simulink model "rfpsc_single"  (R2023b)
settings: Solver=VariableStepAuto  StartTime=0.0  StopTime=.5  RelTol=1e-3
undefined symbols (not defined in the file): f_sw, kpp, L_f, L_g, R_a, R_L, T_s, U_dc, u_gN, w_b, w_g
libraries: simulink x1
settings Model: Creator=maatt  LastModifiedBy=chowd
settings DataIOCC: ReturnWorkspaceOutputs=off

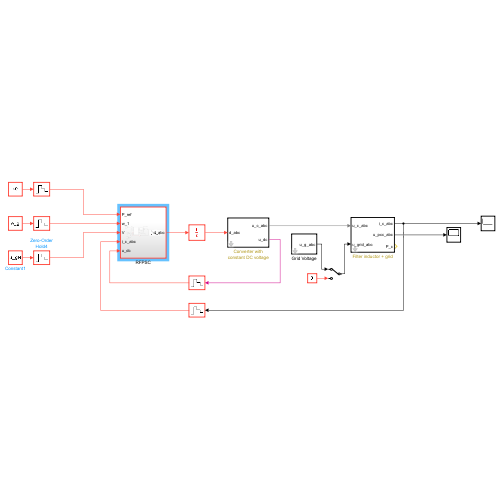
[thumbnail: Simulink's stored preview of the top-level diagram]
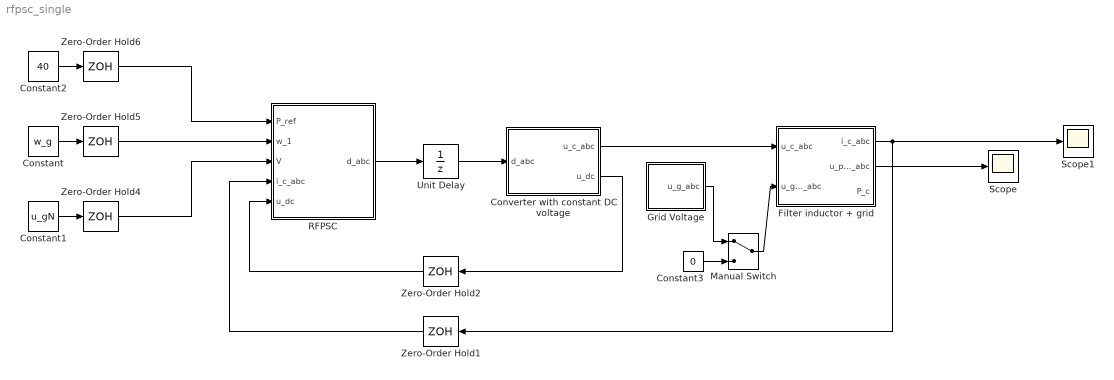
== system rfpsc_single ==
  Constant : Constant  Value=w_g  SampleTime=T_s
  Constant1 : Constant  Value=u_gN  SampleTime=T_s
  Constant2 : Constant  Value=40  SampleTime=T_s
  Constant3 : Constant  Value=0  SampleTime=T_s
  "Converter with constant DC voltage " : Subsystem  mask{f_sw=f_sw, u_dc=U_dc}
      mask prompts: f_sw "Switching frequency (Hz)"; u_dc "DC-bus voltage (V)"
      mask init:
      | T_s = 1/(2*f_sw);
  Filter inductor + grid : Subsystem  mask{L_f=L_f, L_g=L_g, R_L=R_L}
      mask prompts: L_f "Filter inductance (H)"; L_g "Grid inductance (H)"; R_L "Series resistance (ohm)"
  Grid Voltage : Subsystem  mask{U_g=u_gN, angle=0}
      mask prompts: U_g "Phase-voltage"; angle "Shift the phases of voltages"
  Manual Switch : ManualSwitch
  RFPSC : Subsystem
  Scope : Scope
  Scope1 : Scope
  Unit Delay : UnitDelay  SampleTime=T_s  HasFrameUpgradeWarning=on
  Zero-Order Hold{1..2,4..6} (5 alike) : ZeroOrderHold  SampleTime=T_s
  wires:
  "Converter with constant DC voltage "/2(u_dc) -> Zero-Order Hold2/1
  Constant/1 -> Zero-Order Hold5/1
  Constant1/1 -> Zero-Order Hold4/1
  Unit Delay/1 -> "Converter with constant DC voltage "/1(d_abc)
  Zero-Order Hold1/1 -> RFPSC/4(i_c_abc)
  Zero-Order Hold4/1 -> RFPSC/3(V)
  Zero-Order Hold2/1 -> RFPSC/5(u_dc)
  Constant2/1 -> Zero-Order Hold6/1
  Filter inductor + grid/1(i_c_abc) -> Scope1/1, Zero-Order Hold1/1
  Filter inductor + grid/2(u_pcc_abc) -> Scope/1
  Zero-Order Hold6/1 -> RFPSC/1(P_ref)
  Zero-Order Hold5/1 -> RFPSC/2(w_1)
  RFPSC/1(d_abc) -> Unit Delay/1
  Constant3/1 -> Manual Switch/2
  Manual Switch/1 -> Filter inductor + grid/2(u_grid_abc)
  "Converter with constant DC voltage "/1(u_c_abc) -> Filter inductor + grid/1(u_c_abc)
  Grid Voltage/1(u_g_abc) -> Manual Switch/1

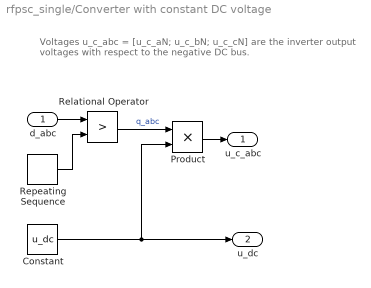
== system rfpsc_single/Converter with constant DC voltage  ==
  note: Voltages u_c_abc = [u_c_aN; u_c_bN; u_c_cN] are the inverter
      | output voltages with respect to the negative DC bus.
  d_abc : Inport
  Constant : Constant  Value=u_dc
  Product : Product
  Relational Operator : RelationalOperator  Operator=>  OutDataTypeStr='double'  InputSameDT=off
  Repeating Sequence : simulink/Sources/Repeating Sequence  rep_seq_t=[0 1 2]*T_s  rep_seq_y=[1 0 1]
  u_c_abc : Outport
  u_dc : Outport  Port=2
  wires:
  Repeating Sequence/1 -> Relational Operator/2
  d_abc/1 -> Relational Operator/1
  Product/1 -> u_c_abc/1
  Relational Operator/1 -> Product/1  "q_abc"
  Constant/1 -> Product/2, u_dc/1

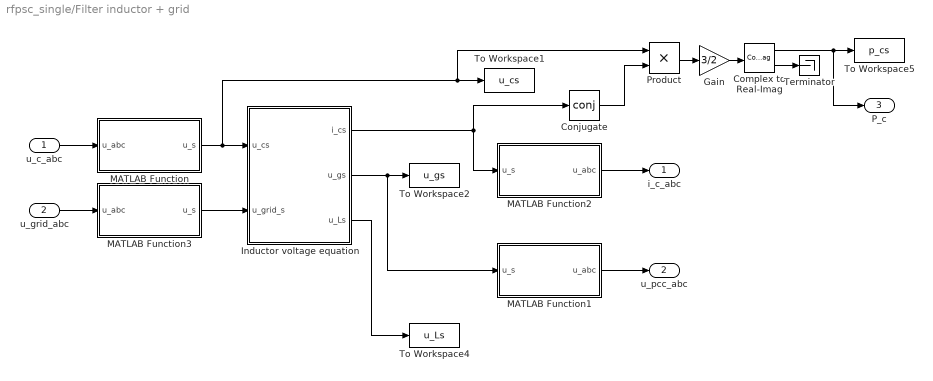
== system rfpsc_single/Filter inductor + grid ==
  u_c_abc : Inport
  u_grid_abc : Inport  Port=2
  Complex to Real-Imag : ComplexToRealImag
  Conjugate : Math  Operator=conj  SignedPower=on  RndMeth=Zero
  Gain : Gain  Gain=3/2
  Inductor voltage equation : Subsystem
  MATLAB Function : MATLAB Function  TreatAsAtomicUnit=on
  MATLAB Function1 : MATLAB Function  TreatAsAtomicUnit=on
  MATLAB Function2 : MATLAB Function  TreatAsAtomicUnit=on
  MATLAB Function3 : MATLAB Function  TreatAsAtomicUnit=on
  Product : Product
  Terminator : Terminator
  To Workspace1 : ToWorkspace  VariableName=u_cs  SaveFormat=Timeseries
  To Workspace2 : ToWorkspace  VariableName=u_gs  SaveFormat=Timeseries
  To Workspace4 : ToWorkspace  VariableName=u_Ls  SaveFormat=Timeseries
  To Workspace5 : ToWorkspace  VariableName=p_cs  SaveFormat=Timeseries
  i_c_abc : Outport
  u_pcc_abc : Outport  Port=2
  P_c : Outport  Port=3
  wires:
  u_c_abc/1 -> MATLAB Function/1(u_abc)
  Inductor voltage equation/1(i_cs) -> MATLAB Function2/1(u_s), Conjugate/1
  MATLAB Function2/1(u_abc) -> i_c_abc/1
  MATLAB Function/1(u_s) -> Inductor voltage equation/1(u_cs), Product/1, To Workspace1/1
  Inductor voltage equation/2(u_gs) -> MATLAB Function1/1(u_s), To Workspace2/1
  Inductor voltage equation/3(u_Ls) -> To Workspace4/1
  MATLAB Function1/1(u_abc) -> u_pcc_abc/1
  Conjugate/1 -> Product/2
  Complex to Real-Imag/1 -> P_c/1, To Workspace5/1
  Complex to Real-Imag/2 -> Terminator/1
  Product/1 -> Gain/1
  Gain/1 -> Complex to Real-Imag/1
  MATLAB Function3/1(u_s) -> Inductor voltage equation/2(u_grid_s)
  u_grid_abc/1 -> MATLAB Function3/1(u_abc)

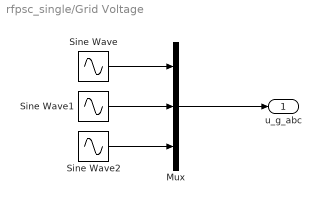
== system rfpsc_single/Grid Voltage ==
  Mux : Mux  Inputs=3
  Sine Wave : Sin  Amplitude=U_g  Frequency=2*pi*50  Phase=pi/2  SampleTime=0
  Sine Wave1 : Sin  Amplitude=U_g  Frequency=2*pi*50  Phase=pi/2 - 2*pi/3  SampleTime=0
  Sine Wave2 : Sin  Amplitude=U_g  Frequency=2*pi*50  Phase=pi/2 - 4*pi/3  SampleTime=0
  u_g_abc : Outport
  wires:
  Mux/1 -> u_g_abc/1
  Sine Wave/1 -> Mux/1
  Sine Wave2/1 -> Mux/3
  Sine Wave1/1 -> Mux/2

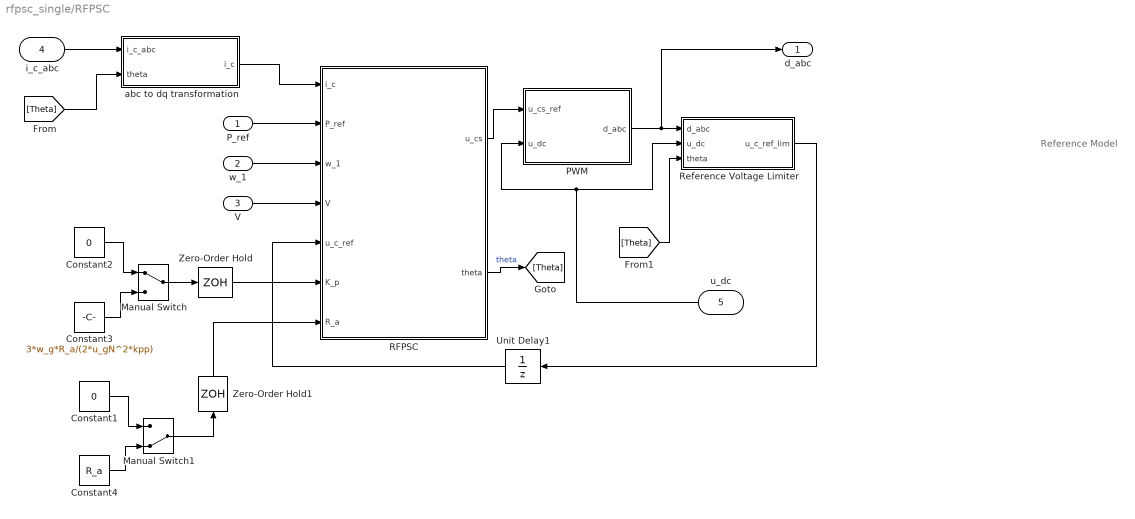
== system rfpsc_single/RFPSC ==
  note: Reference Model
  P_ref : Inport
  w_1 : Inport  Port=2
  V : Inport  Port=3
  i_c_abc : Inport  Port=4
  u_dc : Inport  Port=5
  Constant1 : Constant  Value=0  SampleTime=T_s
  Constant2 : Constant  Value=0  SampleTime=T_s
  Constant3 : Constant  Value=3*w_g*R_a/(2*u_gN^2*kpp)  SampleTime=T_s
  Constant4 : Constant  Value=R_a  SampleTime=T_s
  Manual Switch : ManualSwitch
  Manual Switch1 : ManualSwitch  CurrentSetting=0
  PWM : Subsystem
  RFPSC : Subsystem
  Reference Voltage Limiter : Subsystem
  Unit Delay1 : UnitDelay  SampleTime=-1  HasFrameUpgradeWarning=on
  Zero-Order Hold : ZeroOrderHold  SampleTime=T_s
  Zero-Order Hold1 : ZeroOrderHold  SampleTime=T_s
  abc to dq transformation : MATLAB Function  TreatAsAtomicUnit=on
  d_abc : Outport
  wires:
  w_1/1 -> RFPSC/3(w_1)
  abc to dq transformation/1(i_c) -> RFPSC/1(i_c)
  Unit Delay1/1 -> RFPSC/5(u_c_ref)
  [Theta] -> abc to dq transformation/2(theta)
  [Theta] -> Reference Voltage Limiter/3(theta)
  Reference Voltage Limiter/1(u_c_ref_lim) -> Unit Delay1/1
  P_ref/1 -> RFPSC/2(P_ref)
  i_c_abc/1 -> abc to dq transformation/1(i_c_abc)
  PWM/1(d_abc) -> d_abc/1, Reference Voltage Limiter/1(d_abc)
  V/1 -> RFPSC/4(V)
  u_dc/1 -> PWM/2(u_dc), Reference Voltage Limiter/2(u_dc)
  RFPSC/1(u_cs) -> PWM/1(u_cs_ref)
  RFPSC/2(theta) -> [Theta]  "theta"
  Constant4/1 -> Manual Switch1/2
  Constant2/1 -> Manual Switch/1
  Manual Switch1/1 -> Zero-Order Hold1/1
  Constant1/1 -> Manual Switch1/1
  Constant3/1 -> Manual Switch/2
  Manual Switch/1 -> Zero-Order Hold/1
  Zero-Order Hold/1 -> RFPSC/6(K_p)
  Zero-Order Hold1/1 -> RFPSC/7(R_a)

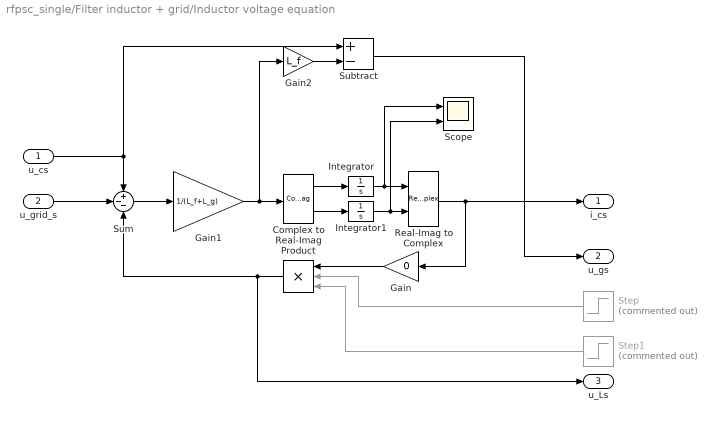
== system rfpsc_single/Filter inductor + grid/Inductor voltage equation ==
  u_cs : Inport
  u_grid_s : Inport  Port=2
  Complex to Real-Imag : ComplexToRealImag
  Gain : Gain  Gain=0
  Gain1 : Gain  Gain=1/(L_f+L_g)
  Gain2 : Gain  Gain=L_f
  Integrator : Integrator
  Integrator1 : Integrator
  Product : Product  Inputs=3
  Real-Imag to Complex : RealImagToComplex
  Scope : Scope  NumInputPorts=2
  Step : Step  Commented=on  Time=0.5  SampleTime=0
  Step1 : Step  Commented=on  Time=0.8  Before=1  After=0  SampleTime=0
  Subtract : Sum  Inputs=+-
  Sum : Sum  Inputs=+--
  i_cs : Outport
  u_gs : Outport  Port=2
  u_Ls : Outport  Port=3
  wires:
  u_cs/1 -> Subtract/1, Sum/1
  Sum/1 -> Gain1/1
  Gain1/1 -> Gain2/1, Complex to Real-Imag/1
  Complex to Real-Imag/1 -> Integrator/1
  Complex to Real-Imag/2 -> Integrator1/1
  Integrator/1 -> Scope/1, Real-Imag to Complex/1
  Integrator1/1 -> Scope/2, Real-Imag to Complex/2
  Real-Imag to Complex/1 -> i_cs/1, Gain/1
  Gain/1 -> Product/1
  Gain2/1 -> Subtract/2
  Subtract/1 -> u_gs/1
  Step/1 -> Product/2
  Product/1 -> Sum/3, u_Ls/1
  Step1/1 -> Product/3
  u_grid_s/1 -> Sum/2

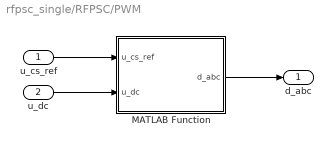
== system rfpsc_single/RFPSC/PWM ==
  u_cs_ref : Inport
  u_dc : Inport  Port=2
  MATLAB Function : MATLAB Function  TreatAsAtomicUnit=on
  d_abc : Outport
  wires:
  u_cs_ref/1 -> MATLAB Function/1(u_cs_ref)
  u_dc/1 -> MATLAB Function/2(u_dc)
  MATLAB Function/1(d_abc) -> d_abc/1

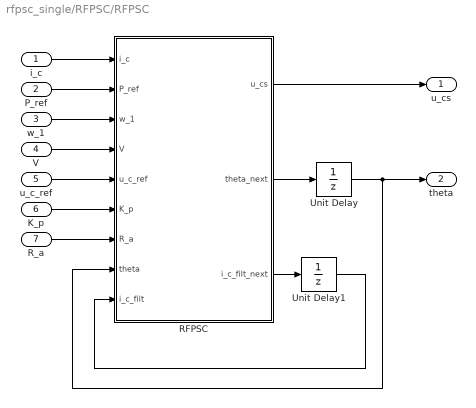
== system rfpsc_single/RFPSC/RFPSC ==
  i_c : Inport
  P_ref : Inport  Port=2
  w_1 : Inport  Port=3
  V : Inport  Port=4
  u_c_ref : Inport  Port=5
  K_p : Inport  Port=6
  R_a : Inport  Port=7
  RFPSC : MATLAB Function  TreatAsAtomicUnit=on  SystemSampleTime=T_s
  Unit Delay : UnitDelay  SampleTime=T_s  HasFrameUpgradeWarning=on
  Unit Delay1 : UnitDelay  SampleTime=T_s  HasFrameUpgradeWarning=on
  u_cs : Outport  OutDataTypeStr=double
      settings: SignalType=complex
  theta : Outport  Port=2  OutDataTypeStr=double
  wires:
  Unit Delay1/1 -> RFPSC/9(i_c_filt)
  RFPSC/3(i_c_filt_next) -> Unit Delay1/1
  Unit Delay/1 -> theta/1, RFPSC/8(theta)
  u_c_ref/1 -> RFPSC/5(u_c_ref)
  w_1/1 -> RFPSC/3(w_1)
  i_c/1 -> RFPSC/1(i_c)
  P_ref/1 -> RFPSC/2(P_ref)
  V/1 -> RFPSC/4(V)
  RFPSC/2(theta_next) -> Unit Delay/1
  RFPSC/1(u_cs) -> u_cs/1
  K_p/1 -> RFPSC/6(K_p)
  R_a/1 -> RFPSC/7(R_a)

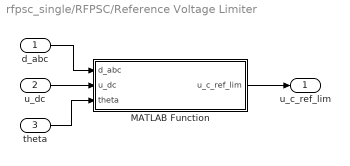
== system rfpsc_single/RFPSC/Reference Voltage Limiter ==
  d_abc : Inport
  u_dc : Inport  Port=2
  theta : Inport  Port=3
  MATLAB Function : MATLAB Function  TreatAsAtomicUnit=on
  u_c_ref_lim : Outport
  wires:
  d_abc/1 -> MATLAB Function/1(d_abc)
  theta/1 -> MATLAB Function/3(theta)
  MATLAB Function/1(u_c_ref_lim) -> u_c_ref_lim/1
  u_dc/1 -> MATLAB Function/2(u_dc)

== matlab function rfpsc_single/Filter inductor + grid/MATLAB Function3 ==
  data: u_abc input size=3; u_s output size=1
function u_s = abc2s(u_abc)

% Space-vector transformation
u_s = 2/3*(u_abc(1) + u_abc(2)*exp(1j*2*pi/3) + u_abc(3)*exp(1j*4*pi/3));

== matlab function rfpsc_single/Filter inductor + grid/MATLAB Function1 ==
  data: u_s input size=1; u_abc output size=3
function u_abc = s2abc(u_s)

% Inverse space-vector transformation
u_abc = real([1; exp(-1j*2*pi/3); exp(-1j*4*pi/3)]*u_s);

== matlab function rfpsc_single/Filter inductor + grid/MATLAB Function ==
  data: u_abc input size=3; u_s output size=1
function u_s = abc2s(u_abc)

% Space-vector transformation
u_s = 2/3*(u_abc(1) + u_abc(2)*exp(1j*2*pi/3) + u_abc(3)*exp(1j*4*pi/3));

== matlab function rfpsc_single/Filter inductor + grid/MATLAB Function2 ==
  data: u_s input size=1; u_abc output size=3
function u_abc = s2abc(u_s)

% Inverse space-vector transformation
u_abc = real([1; exp(-1j*2*pi/3); exp(-1j*4*pi/3)]*u_s);

== matlab function rfpsc_single/RFPSC/PWM/MATLAB Function ==
  data: d_abc output; u_cs_ref input; u_dc input
function d_abc = PWM(u_cs_ref, u_dc)

%% Symmetrical suboscillation PWM
% Components of the voltage space vector
u_c_alpha_ref = real(u_cs_ref);
u_c_beta_ref  = imag(u_cs_ref);

% Phase-voltage references
u_ca_ref = u_c_alpha_ref;
u_cb_ref = .5*(-u_c_alpha_ref + sqrt(3)*u_c_beta_ref);
u_cc_ref = .5*(-u_c_alpha_ref - sqrt(3)*u_c_beta_ref);

% Vector of phase-voltage references
u_c_abc_ref = [u_ca_ref; u_cb_ref; u_cc_ref];

% Symmetrization of the references by adding the zero-sequence voltage
u0 = .5*(max(u_c_abc_ref) + min(u_c_abc_ref));
u_c_abc_ref = u_c_abc_ref - u0;

% Clipping of the reference voltages such that no phase error is caused. 
% If all phase voltage reference are realizable (below u_dc/2), m = 1 holds.
m = max([2*u_c_abc_ref/u_dc; 1]);
u_c_abc_ref = u_c_abc_ref/m;

% Duty cycles, which can be directly used for triangle comparison, 
% if the triangle wave varies between 0...1
d_abc = .5 + u_c_abc_ref/u_dc;

== matlab function rfpsc_single/RFPSC/Reference Voltage Limiter/MATLAB Function ==
  data: d_abc input; u_dc input; u_c_ref_lim output; theta input; w_g parameter; T_s parameter
function u_c_ref_lim = ref_lim(d_abc, u_dc, theta, w_g, T_s)

% % Realized voltage vector is calculated from the clamped duty ratios.
% % If the PWM does not saturate, u_c_ref_lim = u_c_ref holds. The realized
% % voltage vector is needed, e.g., for the current-controller antiwindup.
u_cs_ref_lim = 2/3*(d_abc(1) + d_abc(2)*exp(1j*2*pi/3) ...
    + d_abc(3)*exp(1j*4*pi/3))*u_dc;

% % In estimated rotor flux coordinates
u_c_ref_lim = exp(-1j*(theta + 1.5 * w_g * T_s))*u_cs_ref_lim;

== matlab function rfpsc_single/RFPSC/abc to dq transformation ==
  data: i_c output; i_c_abc input; theta input
function i_c = abc2dq(i_c_abc, theta)

% Space Vector Transformation (abc to alpha-beta)
i_cs = 2/3 * (i_c_abc(1) + i_c_abc(2)*exp(1j*2*pi/3) ... 
    + i_c_abc(3)*exp(1j*4*pi/3));

% Coordinate Transformation (Alpha-beta to dq)
i_c = i_cs * exp(-1j*theta);

== matlab function rfpsc_single/RFPSC/RFPSC/RFPSC ==
  data: i_c input; P_ref input; u_cs output double; theta_next output; w_1 input; V input; u_c_ref input; K_p input; R_a input; theta input; i_c_filt input; T_s parameter; i_c_filt_next output double; w_b parameter; kpp parameter
function [u_cs, theta_next, i_c_filt_next] = ... 
    RFPSC(i_c, P_ref, w_1, V, u_c_ref, K_p, R_a, theta, i_c_filt, ... 
    T_s, w_b, kpp)

% Active power calculation
P = kpp*real(u_c_ref*conj(i_c));

% Equation for grid angular frequency
w_g = w_1;

% Update (integrate) the grid voltage angle
theta_next = theta + T_s * w_g;
if(theta_next > pi)
    theta_next = theta_next - 2*pi;
elseif(theta_next < -pi)
    theta_next = theta_next + 2*pi;
end

% Extracting the real and imaginary values of the complex converter current
i_c_imag = imag(i_c);

% Applying lowpass filter equation to imaginary part of the
% converter current and forming reference current based on power reference
i_c_filt_next =  i_c_filt*(1 - w_b*T_s) + i_c_imag*(w_b*T_s);

if(V == 0 || kpp == 0)
    i_ref = i_c;
else    
    i_ref = P_ref/(V*kpp) + 1j*i_c_filt_next;
end

% Equation for reference voltage
u_c = V;

% Inverse coordinate transformation
u_cs = u_c*exp(1j*(theta + 1.5 * T_s * w_g));
